simulink library "acc"  (R2021b)
settings: Solver=VariableStepAuto  StartTime=0.0  StopTime=10.0  RelTol=1e-3
undefined symbols (not defined in the file or in its folder): AACC_CondensorFanReq_X_enum, AACC_EWP1CCUReq_X_C, AACC_EWP1EDUReq_X_C, AACC_EWP1HVBReq_X_C, AACC_EWP2CCUReq_X_C, AACC_EWP2EDUReq_X_C, AACC_EWP2HVBReq_X_C, AACC_FWV1CCUReq_X_C, AACC_FWV1EDUReq_X_C, AACC_FWV1HVBReq_X_C, AACC_FWV2CCUReq_X_C, AACC_FWV2EDUReq_X_C, AACC_FWV2HVBReq_X_C, AACC_TWVCCUReq_X_C, AACC_TWVEDUReq_X_C, AACC_TWVHVBReq_X_C, ENUM_ACCMODE_CHARGING, ENUM_ACCMODE_COOLING, ENUM_ACCMODE_OFF, ENUM_ACCMODE_SERVICE, ENUM_ACREQ_COOLING, ENUM_ACREQ_NOREQUEST, ENUM_CHILLERINITREQ_NONE, ENUM_CHILLERINITREQ_START, ENUM_CHILLERINITREQ_WAITING, ENUM_CHILLERINITSTA_FINISH, ENUM_CHILLERINITSTA_INPROCESS, ENUM_COOLFANREQ_HI, ENUM_COOLFANREQ_LOW, ENUM_COOLFANREQ_OFF, ENUM_LVBATTSTA_FAIL, ENUM_LVBATTSTA_NORMAL, ENUM_PMMMODE_CHARGE, ENUM_PMMMODE_DRIVE, ENUM_PMMMODE_LVBATCHRG, ENUM_PMMMODE_POWERUP, ENUM_THCMSYS_INACTIVE, FALSE, KACC_CCUFanHighOffTemp_C, KACC_CCUFanHighOnTemp_C, KACC_CCUFanLowOffTemp_C, KACC_CCUFanLowOnTemp_C, KACC_ChillerInitTime_s, KACC_ChillerStartTime_s, KACC_DCDCCalPwrAvailRsv_kW, KACC_EDUFanHighOffTemp_C, KACC_EDUFanHighOnTemp_C, KACC_EDUFanLowOffTemp_C, KACC_EDUFanLowOnTemp_C, KACC_EWP1CalDutyVal_pct, KACC_EWP1CalON_flg, KACC_EWP2CalDutyVal_pct, KACC_EWP2CalON_flg, KACC_EXVCalON_flg, KACC_EXVCalVal_cnt, KACC_FanCalON_flg, KACC_FanCalVal_enum, KACC_FWV1CalON_flg, KACC_FWV1CalVal_flg, KACC_FWV2CalON_flg ... (+51)
libraries: simulink x1
(part 1 of 2)
settings Model: Creator=13615  LastModifiedBy=FVT23131
settings SolverCC: AlgebraicLoopSolver=TrustRegion
settings DataIOCC: SaveFormat=Array  SignalLoggingSaveFormat=ModelDataLogs  ReturnWorkspaceOutputs=off
settings OptimizationCC: BlockReduction=off  BooleanDataType=off
settings DebuggingCC: SaveWithParameterizedLinksMsg=none  UnderspecifiedInitializationDetection=Classic  MergeDetectMultiDrivingBlocksExec=none  SignalResolutionControl=TryResolveAllWithWarning  SFMachineParentedDataDiag=warning  ArithmeticOperatorsInVariantConditions=warning
settings HardwareCC: TargetUnknown=on
settings ModelReferenceCC: PropagateSignalLabelsOutOfModel=off
settings SFSimCC: CustomCodeUndefinedFunction=UseInterfaceOnly
settings ConfigComp: CovMetricSettings=dw  CovSaveCumulativeToWorkspaceVar=on  CovSaveSingleToWorkspaceVar=on

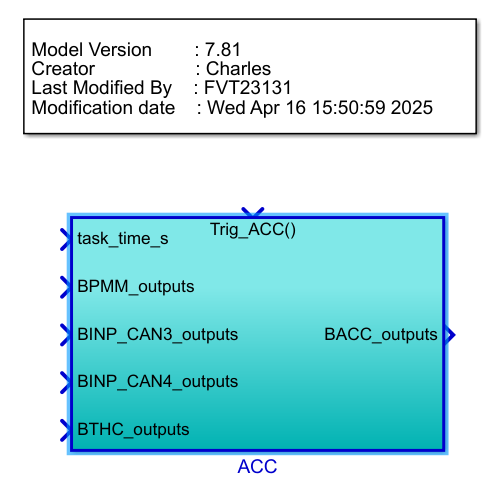
[thumbnail: Simulink's stored preview of the top-level diagram]
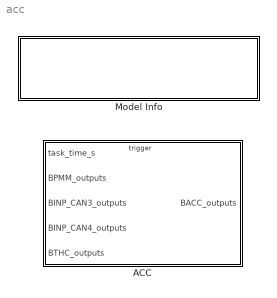
== system acc ==
  ACC : Subsystem  TreatAsAtomicUnit=on
      settings: RTWSystemCode=Nonreusable function  RTWFcnNameOpts=Use subsystem name  RTWFileNameOpts=Use subsystem name
  Model Info : Subsystem  LoadFcn=slcm LoadBlock;  InitFcn=slcm('UpdateAllCMBlocksInThisModelInit')  mask(CMBlock){InitialSaveTempField=, InitialBlockCM=None, BlockCM=None, Frame=on, SaveTempField=, DisplayStringWithTags=|, MaskDisplayString=Model Version        : 7.84\nCreator                   : Charles\nLast Modified By    : FVT23131\nModification date    : Wed Apr 16 17:01:18 2025, HorizontalTextAlignment=Left, LeftAlignmentValue=0.02, SourceBlockDiagram=acc, TagMaxNumber=20, CMTag1=, CMTag2=, CMTag3=, CMTag4=, CMTag5=, CMTag6=, CMTag7=, CMTag8=, CMTag9=, CMTag10=, CMTag11=, CMTag12=, CMTag13=, CMTag14=, CMTag15=, CMTag16=, CMTag17=, CMTag18=, CMTag19=, CMTag20=}
      mask DisplayStringWithTags=|
      | Model Version        : %<ModelVersion>
      | Creator                   : Charles
      | Last Modified By    : %<LastModifiedBy>
      | Modification date    : %<LastModificationDate>
      mask help: This block allows revision control information to be displayed within the model.
      settings: CopyFcn=slcm CopyBlock;  DeleteFcn=slcm Cancel;  PostSaveFcn=slcm('UpdateAllCMBlocksInThisModel')  NameChangeFcn=slcm Rename;  OpenFcn=slcm
      mask Display: text(str2num(LeftAlignmentValue), 0.5, MaskDisplayString, 'HorizontalAlignment', HorizontalTextAlignment)

== system acc/ACC ==
  task_time_s : Inport
  BPMM_outputs : Inport  Port=2  OutDataTypeStr=Bus: BPMM_outputs
  BINP_CAN3_outputs : Inport  Port=3  OutDataTypeStr=Bus: BINP_CAN3_outputs
  BINP_CAN4_outputs : Inport  Port=4  OutDataTypeStr=Bus: BINP_CAN4_outputs
  BTHC_outputs : Inport  Port=5  OutDataTypeStr=Bus: BTHC_outputs
  Trig_ACC : TriggerPort  TriggerType=function-call  VariantControl=(inherit)
  ACC : Subsystem  Commented=on  AncestorBlock=acc/ACC/ACC
  Bus Creator : BusCreator  Inputs=4  OutDataTypeStr=Bus: BACC_outputs
  Bus Selector : BusSelector  OutputSignals=VINP_COMPActualPwr_W
  Bus Selector1 : BusSelector  OutputSignals=VINP_LVBattDet12V_V,VINP_HVBPwrAvailDchrg_kW,VINP_FrMCUDCBusVolt_V,VINP_FrMCUDCBusCurr_A,VINP_RrMCUDCBusVolt_V,VINP_RrMCUDCBusCurr_A,VINP_DCDCHVCur_A,VINP_DCDCInVoltInf_V
  Bus Selector12 : BusSelector  OutputSignals=VTHC_FDFrLeAPTCHeatPwrCmd_W,VTHC_FDFrRiAPTCHeatPwrCmd_W,VTHC_FDRrAPTCHeatPwrCmd_W,VTHC_FDFrWPTCHeatPwrCmd_W
  Bus Selector2 : BusSelector  OutputSignals=VPMM_HVPwrSta_flg,VPMM_LVPwrSta_flg
  Model Info : simulink/Model-Wide Utilities/Model Info  Frame=on  DisplayStringWithTags=|  HorizontalTextAlignment=Center  LeftAlignmentValue=0.5
      | $Id: ACC.mdl 2018-05-29 Lon $
      | Modified By %<ModifiedBy>
      | Modified Date : %<ModifiedDate>
  THCM : Subsystem
  BACC_outputs : Outport  OutDataTypeStr=Bus: BACC_outputs  VectorParamsAs1DForOutWhenUnconnected=off
  wires:
  BPMM_outputs/1 -> Bus Selector2/1
  Bus Creator/1 -> BACC_outputs/1  "BACC_outputs"
  BINP_CAN3_outputs/1 -> Bus Selector1/1
  Bus Selector1/1 -> THCM/4(VINP_LVBattDet12V_V)  "<VINP_LVBattDet12V_V>"
  task_time_s/1 -> THCM/1(task_time_s)
  Bus Selector1/2 -> THCM/5(VINP_HVBPwrAvailDchrg_kW)  "<VINP_HVBPwrAvailDchrg_kW>"
  Bus Selector1/3 -> THCM/6(VINP_FrMCUDCBusVolt_V)  "<VINP_FrMCUDCBusVolt_V>"
  Bus Selector1/4 -> THCM/7(VINP_FrMCUDCBusCurr_A)  "<VINP_FrMCUDCBusCurr_A>"
  Bus Selector1/5 -> THCM/8(VINP_RrMCUDCBusVolt_V)  "<VINP_RrMCUDCBusVolt_V>"
  Bus Selector1/6 -> THCM/9(VINP_RrMCUDCBusCurr_A)  "<VINP_RrMCUDCBusCurr_A>"
  THCM/3(VACC_VehHVPwrAvail4THCM_W) -> Bus Creator/3
  THCM/1(VACC_HVTHCMSysAvail_enum) -> Bus Creator/1
  THCM/2(VACC_LVBattVoltSta_enum) -> Bus Creator/2
  Bus Selector2/1 -> THCM/2(VPMM_HVPwrSta_flg)  "<VPMM_HVPwrSta_flg>"
  Bus Selector2/2 -> THCM/3(VPMM_LVPwrSta_flg)  "<VPMM_LVPwrSta_flg>"
  Bus Selector1/7 -> THCM/10(VINP_DCDCHVCur_A)  "<VINP_DCDCHVCur_A>"
  Bus Selector1/8 -> THCM/11(VINP_DCDCInVoltInf_V)  "<VINP_DCDCInVoltInf_V>"
  BINP_CAN4_outputs/1 -> Bus Selector/1
  Bus Selector/1 -> THCM/12(VINP_COMPActualPwr_W)  "<VINP_COMPActualPwr_W>"
  BTHC_outputs/1 -> Bus Selector12/1
  Bus Selector12/1 -> THCM/13(VTHC_FDFrLeAPTCHeatPwrCmd_W)  "<VTHC_FDFrLeAPTCHeatPwrCmd_W>"
  Bus Selector12/2 -> THCM/14(VTHC_FDFrRiAPTCHeatPwrCmd_W)  "<VTHC_FDFrRiAPTCHeatPwrCmd_W>"
  Bus Selector12/3 -> THCM/15(VTHC_FDRrAPTCHeatPwrCmd_W)  "<VTHC_FDRrAPTCHeatPwrCmd_W>"
  Bus Selector12/4 -> THCM/16(VTHC_FDFrWPTCHeatPwrCmd_W)  "<VTHC_FDFrWPTCHeatPwrCmd_W>"
  THCM/4(VACC_TMPwrAvailDchrg_kW) -> Bus Creator/4

== system acc/Model Info ==
  EmptySubsystem : Subsystem

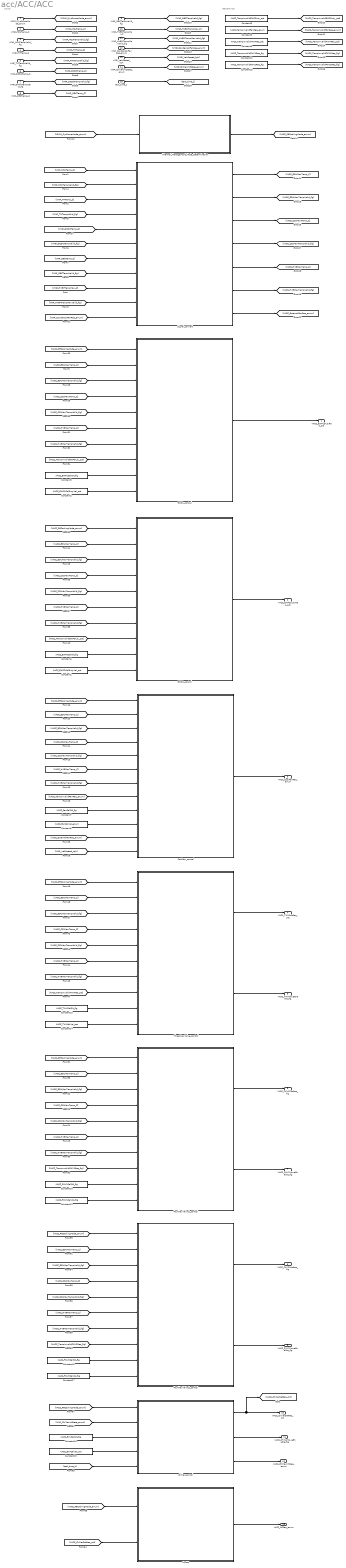
== system acc/ACC/ACC ==
  note: General Cal
  note: Inputs
  VPMM_SysPowerMode_enum : Inport
  VINP_MCUTemp_C : Inport  Port=2
  VINP_MCUTempValid_flg : Inport  Port=3
  VINP_TMTemp_C : Inport  Port=4
  VINP_TMTempValid_flg : Inport  Port=5
  VINP_DCDCTemp_C : Inport  Port=6
  VINP_DCDCTempValid_flg : Inport  Port=7
  VINP_OBCTemp_C : Inport  Port=8
  VINP_OBCTempValid_flg : Inport  Port=9
  VINP_HVBMTempMax_C : Inport  Port=10
  VINP_HVBMTempMaxValid_flg : Inport  Port=11
  VINP_CondensorFanReq_enum : Inport  Port=12
  VINP_VehSpeed_kph : Inport  Port=13
  VINP_ChillerInitState_enum : Inport  Port=14
  task_time_s : Inport  Port=15
  ACReq : Subsystem
  Chiller_control : Subsystem
  Constant1 : Constant  Value=KACC_EWP2CalDutyVal_pct
  Constant10 : Constant  Value=KACC_FWV1CalON_flg
  Constant11 : Constant  Value=KACC_FWV1CalVal_flg
  Constant12 : Constant  Value=KACC_TempInvalidFWV1Req_flg
  Constant13 : Constant  Value=KACC_TWVCalON_flg
  Constant14 : Constant  Value=KACC_TWVCalVal_pct
  Constant15 : Constant  Value=KACC_TempInvalidFWV2Req_flg
  Constant16 : Constant  Value=KACC_FWV2CalON_flg
  Constant17 : Constant  Value=KACC_FWV2CalVal_flg
  Constant18 : Constant  Value=KACC_EXVCalON_flg
  Constant19 : Constant  Value=KACC_EXVCalVal_cnt
  Constant2 : Constant  Value=KACC_EWP1CalDutyVal_pct
  Constant3 : Constant  Value=KACC_EWP1CalON_flg
  Constant4 : Constant  Value=KACC_EWP2CalON_flg
  Constant5 : Constant  Value=KACC_TempInvalidEWPDuty_pct
  Constant6 : Constant  Value=KACC_FanCalVal_enum
  Constant7 : Constant  Value=KACC_FanCalON_flg
  Constant8 : Constant  Value=KACC_TempInvalidTWVReq_pct
  Constant9 : Constant  Value=KACC_TempInvalidFanReq_enum
  CoolFan_control : Subsystem
  EWP1_control : Subsystem
  EWP2_control : Subsystem
  FourWayValve1_control : Subsystem
  FourWayValve2_control : Subsystem
  Signal_convert : Subsystem
  Thermal_Managemant_Mode_Determination : Subsystem
  ThreeWayValve_control : Subsystem
  VACC_EWP1DutyReq_pct : Outport  VectorParamsAs1DForOutWhenUnconnected=off
  VACC_EWP2DutyReq_pct : Outport  Port=2  VectorParamsAs1DForOutWhenUnconnected=off
  VACC_CoolFanReq_enum : Outport  Port=3  VectorParamsAs1DForOutWhenUnconnected=off
  VACC_TWVPosReq_pct : Outport  Port=4  VectorParamsAs1DForOutWhenUnconnected=off
  VACC_TWVMoveEnable_flg : Outport  Port=5  VectorParamsAs1DForOutWhenUnconnected=off
  VACC_FWV1PosReq_flg : Outport  Port=6  VectorParamsAs1DForOutWhenUnconnected=off
  VACC_FWV1MoveEnable_flg : Outport  Port=7  VectorParamsAs1DForOutWhenUnconnected=off
  VACC_FWV2PosReq_flg : Outport  Port=8  VectorParamsAs1DForOutWhenUnconnected=off
  VACC_FWV2MoveEnable_flg : Outport  Port=9  VectorParamsAs1DForOutWhenUnconnected=off
  VACC_ChillerSetReq_cnt : Outport  Port=10  VectorParamsAs1DForOutWhenUnconnected=off
  VACC_ChillerMoveEnable_flg : Outport  Port=11  VectorParamsAs1DForOutWhenUnconnected=off
  VACC_ChillerInitReq_enum : Outport  Port=12  VectorParamsAs1DForOutWhenUnconnected=off
  VACC_ACReq_enum : Outport  Port=13  VectorParamsAs1DForOutWhenUnconnected=off
  wires:
  [task_time_s] -> Chiller_control/5(task_time_s)
  task_time_s/1 -> [task_time_s]
  [VINP_ChillerInitState_enum] -> Chiller_control/2(VINP_ChillerInitState_enum)
  VINP_ChillerInitState_enum/1 -> [VINP_ChillerInitState_enum]
  Chiller_control/3(VACC_ChillerInitReq_enum) -> VACC_ChillerInitReq_enum/1  "VACC_ChillerInitReq_enum"
  Chiller_control/1(VACC_ChillerSetReq_cnt) -> [VACC_ChillerSetReq_cnt], VACC_ChillerSetReq_cnt/1  "VACC_ChillerSetReq_cnt"
  [VACC_PECoolingMode_enum] -> Chiller_control/1(VACC_PECoolingMode_enum)
  Constant18/1 -> Chiller_control/3(KACC_EXVCalON_flg)  "KACC_EXVCalON_flg"
  Constant19/1 -> Chiller_control/4(KACC_EXVCalVal_cnt)  "KACC_EXVCalVal_cnt"
  Chiller_control/2(VACC_ChillerMoveEnable_flg) -> VACC_ChillerMoveEnable_flg/1  "VACC_ChillerMoveEnable_flg"
  FourWayValve2_control/2(VACC_FWV2MoveEnable_flg) -> VACC_FWV2MoveEnable_flg/1  "VACC_FWV2MoveEnable_flg"
  Constant17/1 -> FourWayValve2_control/10(KACC_FWV2CalVal_flg)  "KACC_FWV2CalVal_flg"
  Constant16/1 -> FourWayValve2_control/9(KACC_FWV2CalON_flg)  "KACC_FWV2CalON_flg"
  [VACC_PECoolingMode_enum] -> FourWayValve2_control/1(VACC_PECoolingMode_enum)
  [VACC_CCUMaxTempValid_flg] -> FourWayValve2_control/5(VACC_CCUMaxTempValid_flg)
  [VACC_CCUMaxTemp_C] -> FourWayValve2_control/4(VACC_CCUMaxTemp_C)
  [VACC_EDUMaxTemp_C] -> FourWayValve2_control/2(VACC_EDUMaxTemp_C)
  [VACC_EDUMaxTempValid_flg] -> FourWayValve2_control/3(VACC_EDUMaxTempValid_flg)
  [VACC_HVBMaxTempValid_flg] -> FourWayValve2_control/7(VACC_HVBMaxTempValid_flg)
  FourWayValve2_control/1(VACC_FWV2PosReq_flg) -> VACC_FWV2PosReq_flg/1  "VACC_FWV2PosReq_flg"
  [VACC_HVBMaxTemp_C] -> FourWayValve2_control/6(VACC_HVBMaxTemp_C)
  [KACC_TempInvalidFWV2Req_flg] -> FourWayValve2_control/8(KACC_TempInvalidFWV2Req_flg)
  [KACC_TempInvalidFWV1Req_flg] -> FourWayValve1_control/8(KACC_TempInvalidFWV1Req_flg)
  [KACC_TempInvalidTWVReq_pct] -> ThreeWayValve_control/8(KACC_TempInvalidTWVReq_pct)
  Constant15/1 -> [KACC_TempInvalidFWV2Req_flg]  "KACC_TempInvalidFWV2Req_flg"
  Constant12/1 -> [KACC_TempInvalidFWV1Req_flg]  "KACC_TempInvalidFWV1Req_flg"
  [VACC_HVBMaxTemp_C] -> FourWayValve1_control/6(VACC_HVBMaxTemp_C)
  FourWayValve1_control/1(VACC_FWV1PosReq_flg) -> VACC_FWV1PosReq_flg/1  "VACC_FWV1PosReq_flg"
  [VACC_HVBMaxTempValid_flg] -> FourWayValve1_control/7(VACC_HVBMaxTempValid_flg)
  [VACC_EDUMaxTempValid_flg] -> FourWayValve1_control/3(VACC_EDUMaxTempValid_flg)
  [VACC_EDUMaxTemp_C] -> FourWayValve1_control/2(VACC_EDUMaxTemp_C)
  [VACC_CCUMaxTemp_C] -> FourWayValve1_control/4(VACC_CCUMaxTemp_C)
  [VACC_CCUMaxTempValid_flg] -> FourWayValve1_control/5(VACC_CCUMaxTempValid_flg)
  [VACC_PECoolingMode_enum] -> FourWayValve1_control/1(VACC_PECoolingMode_enum)
  Constant10/1 -> FourWayValve1_control/9(KACC_FWV1CalON_flg)  "KACC_FWV1CalON_flg"
  Constant11/1 -> FourWayValve1_control/10(KACC_FWV1CalVal_flg)  "KACC_FWV1CalVal_flg"
  FourWayValve1_control/2(VACC_FWV1MoveEnable_flg) -> VACC_FWV1MoveEnable_flg/1  "VACC_FWV1MoveEnable_flg"
  ThreeWayValve_control/2(VACC_TWVMoveEnable_flg) -> VACC_TWVMoveEnable_flg/1  "VACC_TWVMoveEnable_flg"
  Constant14/1 -> ThreeWayValve_control/10(KACC_TWVCalVal_pct)  "KACC_TWVCalVal_pct"
  Constant13/1 -> ThreeWayValve_control/9(KACC_TWVCalON_flg)  "KACC_TWVCalON_flg"
  Constant8/1 -> [KACC_TempInvalidTWVReq_pct]  "KACC_TempInvalidTWVReq_pct"
  [VACC_PECoolingMode_enum] -> ThreeWayValve_control/1(VACC_PECoolingMode_enum)
  [VACC_CCUMaxTempValid_flg] -> ThreeWayValve_control/5(VACC_CCUMaxTempValid_flg)
  [VACC_CCUMaxTemp_C] -> ThreeWayValve_control/4(VACC_CCUMaxTemp_C)
  [VACC_EDUMaxTemp_C] -> ThreeWayValve_control/2(VACC_EDUMaxTemp_C)
  [VACC_EDUMaxTempValid_flg] -> ThreeWayValve_control/3(VACC_EDUMaxTempValid_flg)
  [VACC_HVBMaxTempValid_flg] -> ThreeWayValve_control/7(VACC_HVBMaxTempValid_flg)
  ThreeWayValve_control/1(VACC_TWVPosReq_pct) -> VACC_TWVPosReq_pct/1  "VACC_TWVPosReq_pct"
  [VACC_HVBMaxTemp_C] -> ThreeWayValve_control/6(VACC_HVBMaxTemp_C)
  [VINP_VehSpeed_kph] -> CoolFan_control/12(VINP_VehSpeed_kph)
  VINP_VehSpeed_kph/1 -> [VINP_VehSpeed_kph]
  [VACC_ExternalFanReq_enum] -> CoolFan_control/11(VACC_ExternalFanReq_enum)
  Signal_convert/7(VACC_ExternalFanReq_enum) -> [VACC_ExternalFanReq_enum]  "VACC_ExternalFanReq_enum"
  [VINP_CondensorFanReq_enum] -> Signal_convert/11(VINP_CondensorFanReq_enum)
  [KACC_TempInvalidFanReq_enum] -> CoolFan_control/8(KACC_TempInvalidFanReq_enum)
  Constant6/1 -> CoolFan_control/10(KACC_FanCalVal_enum)  "KACC_FanCalVal_enum"
  Constant7/1 -> CoolFan_control/9(KACC_FanCalON_flg)  "KACC_FanCalON_flg"
  [VACC_CCUMaxTemp_C] -> CoolFan_control/4(VACC_CCUMaxTemp_C)
  [VACC_EDUMaxTempValid_flg] -> CoolFan_control/3(VACC_EDUMaxTempValid_flg)
  [VACC_EDUMaxTemp_C] -> CoolFan_control/2(VACC_EDUMaxTemp_C)
  [VACC_HVBMaxTempValid_flg] -> CoolFan_control/7(VACC_HVBMaxTempValid_flg)
  [VACC_HVBMaxTemp_C] -> CoolFan_control/6(VACC_HVBMaxTemp_C)
  [VACC_CCUMaxTempValid_flg] -> CoolFan_control/5(VACC_CCUMaxTempValid_flg)
  [VACC_PECoolingMode_enum] -> CoolFan_control/1(VACC_PECoolingMode_enum)
  CoolFan_control/1(VACC_CoolFanReq_enum) -> VACC_CoolFanReq_enum/1  "VACC_CoolFanReq_enum"
  EWP2_control/1(VACC_EWP2DutyReq_pct) -> VACC_EWP2DutyReq_pct/1  "VACC_EWP2DutyReq_pct"
  [VACC_PECoolingMode_enum] -> EWP2_control/1(VACC_PECoolingMode_enum)
  [VACC_CCUMaxTempValid_flg] -> EWP2_control/5(VACC_CCUMaxTempValid_flg)
  [VACC_HVBMaxTemp_C] -> EWP2_control/6(VACC_HVBMaxTemp_C)
  [VACC_HVBMaxTempValid_flg] -> EWP2_control/7(VACC_HVBMaxTempValid_flg)
  [VACC_EDUMaxTemp_C] -> EWP2_control/2(VACC_EDUMaxTemp_C)
  [VACC_EDUMaxTempValid_flg] -> EWP2_control/3(VACC_EDUMaxTempValid_flg)
  [VACC_CCUMaxTemp_C] -> EWP2_control/4(VACC_CCUMaxTemp_C)
  [KACC_TempInvalidEWPDuty_pct] -> EWP2_control/8(KACC_TempInvalidEWPDuty_pct)
  Constant4/1 -> EWP2_control/9(KACC_EWP2CalON_flg)  "KACC_EWP2CalON_flg"
  Constant1/1 -> EWP2_control/10(KACC_EWP2CalDutyVal_pct)  "KACC_EWP2CalDutyVal_pct"
  Constant2/1 -> EWP1_control/10(KACC_EWP1CalDutyVal_pct)  "KACC_EWP1CalDutyVal_pct"
  Constant3/1 -> EWP1_control/9(KACC_EWP1CalON_flg)  "KACC_EWP1CalON_flg"
  [KACC_TempInvalidEWPDuty_pct] -> EWP1_control/8(KACC_TempInvalidEWPDuty_pct)
  [VACC_CCUMaxTemp_C] -> EWP1_control/4(VACC_CCUMaxTemp_C)
  [VACC_EDUMaxTempValid_flg] -> EWP1_control/3(VACC_EDUMaxTempValid_flg)
  [VACC_EDUMaxTemp_C] -> EWP1_control/2(VACC_EDUMaxTemp_C)
  [VACC_HVBMaxTempValid_flg] -> EWP1_control/7(VACC_HVBMaxTempValid_flg)
  [VACC_HVBMaxTemp_C] -> EWP1_control/6(VACC_HVBMaxTemp_C)
  [VACC_CCUMaxTempValid_flg] -> EWP1_control/5(VACC_CCUMaxTempValid_flg)
  [VACC_PECoolingMode_enum] -> EWP1_control/1(VACC_PECoolingMode_enum)
  Constant9/1 -> [KACC_TempInvalidFanReq_enum]  "KACC_TempInvalidFanReq_enum"
  Constant5/1 -> [KACC_TempInvalidEWPDuty_pct]  "KACC_TempInvalidEWPDuty_pct"
  Signal_convert/4(VACC_CCUMaxTempValid_flg) -> [VACC_CCUMaxTempValid_flg]  "VACC_CCUMaxTempValid_flg"
  Signal_convert/5(VACC_HVBMaxTemp_C) -> [VACC_HVBMaxTemp_C]  "VACC_HVBMaxTemp_C"
  Signal_convert/3(VACC_CCUMaxTemp_C) -> [VACC_CCUMaxTemp_C]  "VACC_CCUMaxTemp_C"
  Signal_convert/6(VACC_HVBMaxTempValid_flg) -> [VACC_HVBMaxTempValid_flg]  "VACC_HVBMaxTempValid_flg"
  Signal_convert/2(VACC_EDUMaxTempValid_flg) -> [VACC_EDUMaxTempValid_flg]  "VACC_EDUMaxTempValid_flg"
  Signal_convert/1(VACC_EDUMaxTemp_C) -> [VACC_EDUMaxTemp_C]  "VACC_EDUMaxTemp_C"
  [VINP_HVBMTempMaxValid_flg] -> Signal_convert/10(VINP_HVBMTempMaxValid_flg)
  [VINP_HVBMTempMax_C] -> Signal_convert/9(VINP_HVBMTempMax_C)
  [VINP_OBCTempValid_flg] -> Signal_convert/8(VINP_OBCTempValid_flg)
  [VINP_OBCTemp_C] -> Signal_convert/7(VINP_OBCTemp_C)
  [VINP_MCUTemp_C] -> Signal_convert/1(VINP_MCUTemp_C)
  [VINP_DCDCTempValid_flg] -> Signal_convert/6(VINP_DCDCTempValid_flg)
  [VINP_MCUTempValid_flg] -> Signal_convert/2(VINP_MCUTempValid_flg)
  [VINP_TMTemp_C] -> Signal_convert/3(VINP_TMTemp_C)
  [VINP_TMTempValid_flg] -> Signal_convert/4(VINP_TMTempValid_flg)
  [VINP_DCDCTemp_C] -> Signal_convert/5(VINP_DCDCTemp_C)
  VINP_CondensorFanReq_enum/1 -> [VINP_CondensorFanReq_enum]
  VINP_DCDCTemp_C/1 -> [VINP_DCDCTemp_C]
  VINP_TMTemp_C/1 -> [VINP_TMTemp_C]
  VINP_MCUTemp_C/1 -> [VINP_MCUTemp_C]
  VPMM_SysPowerMode_enum/1 -> [VPMM_SysPowerMode_enum]
  VINP_OBCTemp_C/1 -> [VINP_OBCTemp_C]
  VINP_HVBMTempMax_C/1 -> [VINP_HVBMTempMax_C]
  VINP_MCUTempValid_flg/1 -> [VINP_MCUTempValid_flg]
  VINP_TMTempValid_flg/1 -> [VINP_TMTempValid_flg]
  VINP_DCDCTempValid_flg/1 -> [VINP_DCDCTempValid_flg]
  VINP_OBCTempValid_flg/1 -> [VINP_OBCTempValid_flg]
  VINP_HVBMTempMaxValid_flg/1 -> [VINP_HVBMTempMaxValid_flg]
  Thermal_Managemant_Mode_Determination/1(VACC_PECoolingMode_enum) -> [VACC_PECoolingMode_enum]
  [VPMM_SysPowerMode_enum] -> Thermal_Managemant_Mode_Determination/1(VPMM_SysPowerMode_enum)
  EWP1_control/1(VACC_EWP1DutyReq_pct) -> VACC_EWP1DutyReq_pct/1  "VACC_EWP1DutyReq_pct"
  [VACC_ChillerSetReq_cnt] -> ACReq/2(VACC_ChillerSetReq_cnt)
  [VACC_PECoolingMode_enum] -> ACReq/1(VACC_PECoolingMode_enum)
  ACReq/1(VACC_ACReq_enum) -> VACC_ACReq_enum/1  "VACC_ACReq_enum"

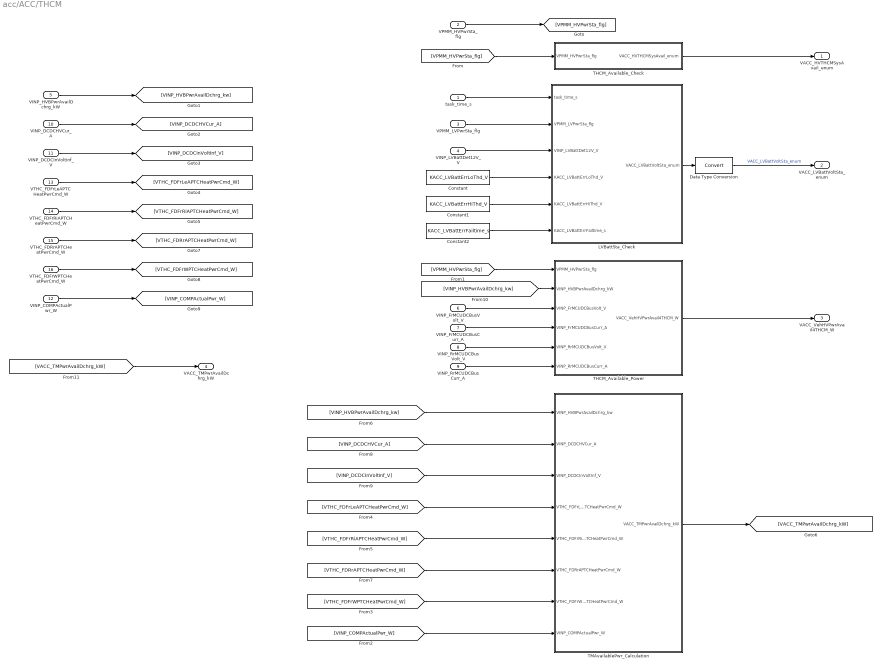
== system acc/ACC/THCM ==
  task_time_s : Inport
  VPMM_HVPwrSta_flg : Inport  Port=2
  VPMM_LVPwrSta_flg : Inport  Port=3
  VINP_LVBattDet12V_V : Inport  Port=4
  VINP_HVBPwrAvailDchrg_kW : Inport  Port=5
  VINP_FrMCUDCBusVolt_V : Inport  Port=6
  VINP_FrMCUDCBusCurr_A : Inport  Port=7
  VINP_RrMCUDCBusVolt_V : Inport  Port=8
  VINP_RrMCUDCBusCurr_A : Inport  Port=9
  VINP_DCDCHVCur_A : Inport  Port=10
  VINP_DCDCInVoltInf_V : Inport  Port=11
  VINP_COMPActualPwr_W : Inport  Port=12
  VTHC_FDFrLeAPTCHeatPwrCmd_W : Inport  Port=13
  VTHC_FDFrRiAPTCHeatPwrCmd_W : Inport  Port=14
  VTHC_FDRrAPTCHeatPwrCmd_W : Inport  Port=15
  VTHC_FDFrWPTCHeatPwrCmd_W : Inport  Port=16
  Constant : Constant  Value=KACC_LVBattErrLoThd_V
  Constant1 : Constant  Value=KACC_LVBattErrHiThd_V
  Constant2 : Constant  Value=KACC_LVBattErrFailtime_s
  Data Type Conversion : DataTypeConversion
  LVBattSta_Check : Stateflow chart  TreatAsAtomicUnit=on
  THCM_Available_Check : Subsystem
  THCM_Available_Power : Subsystem
  TMAvailablePwr_Calculation : Subsystem
  VACC_HVTHCMSysAvail_enum : Outport
  VACC_LVBattVoltSta_enum : Outport  Port=2
  VACC_VehHVPwrAvail4THCM_W : Outport  Port=3
  VACC_TMPwrAvailDchrg_kW : Outport  Port=4
  wires:
  VINP_LVBattDet12V_V/1 -> LVBattSta_Check/3(VINP_LVBattDet12V_V)
  Constant/1 -> LVBattSta_Check/4(KACC_LVBattErrLoThd_V)
  Constant1/1 -> LVBattSta_Check/5(KACC_LVBattErrHiThd_V)
  Constant2/1 -> LVBattSta_Check/6(KACC_LVBattErrFailtime_s)
  LVBattSta_Check/1(VACC_LVBattVoltSta_enum) -> Data Type Conversion/1
  task_time_s/1 -> LVBattSta_Check/1(task_time_s)
  VPMM_HVPwrSta_flg/1 -> [VPMM_HVPwrSta_flg]
  Data Type Conversion/1 -> VACC_LVBattVoltSta_enum/1  "VACC_LVBattVoltSta_enum"
  VPMM_LVPwrSta_flg/1 -> LVBattSta_Check/2(VPMM_LVPwrSta_flg)
  [VPMM_HVPwrSta_flg] -> THCM_Available_Check/1(VPMM_HVPwrSta_flg)
  THCM_Available_Check/1(VACC_HVTHCMSysAvail_enum) -> VACC_HVTHCMSysAvail_enum/1
  [VPMM_HVPwrSta_flg] -> THCM_Available_Power/1(VPMM_HVPwrSta_flg)
  THCM_Available_Power/1(VACC_VehHVPwrAvail4THCM_W) -> VACC_VehHVPwrAvail4THCM_W/1
  VINP_FrMCUDCBusVolt_V/1 -> THCM_Available_Power/3(VINP_FrMCUDCBusVolt_V)
  VINP_FrMCUDCBusCurr_A/1 -> THCM_Available_Power/4(VINP_FrMCUDCBusCurr_A)
  VINP_RrMCUDCBusVolt_V/1 -> THCM_Available_Power/5(VINP_RrMCUDCBusVolt_V)
  VINP_RrMCUDCBusCurr_A/1 -> THCM_Available_Power/6(VINP_RrMCUDCBusCurr_A)
  [VINP_HVBPwrAvailDchrg_kw] -> THCM_Available_Power/2(VINP_HVBPwrAvailDchrg_kW)
  [VINP_HVBPwrAvailDchrg_kw] -> TMAvailablePwr_Calculation/1(VINP_HVBPwrAvailDchrg_kw)
  TMAvailablePwr_Calculation/1(VACC_TMPwrAvailDchrg_kW) -> [VACC_TMPwrAvailDchrg_kW]
  [VTHC_FDFrWPTCHeatPwrCmd_W] -> TMAvailablePwr_Calculation/7(VTHC_FDFrWPTCHeatPwrCmd_W)
  [VTHC_FDRrAPTCHeatPwrCmd_W] -> TMAvailablePwr_Calculation/6(VTHC_FDRrAPTCHeatPwrCmd_W)
  [VTHC_FDFrLeAPTCHeatPwrCmd_W] -> TMAvailablePwr_Calculation/4(VTHC_FDFrLeAPTCHeatPwrCmd_W)
  [VINP_DCDCInVoltInf_V] -> TMAvailablePwr_Calculation/3(VINP_DCDCInVoltInf_V)
  [VTHC_FDFrRiAPTCHeatPwrCmd_W] -> TMAvailablePwr_Calculation/5(VTHC_FDFrRiAPTCHeatPwrCmd_W)
  [VINP_COMPActualPwr_W] -> TMAvailablePwr_Calculation/8(VINP_COMPActualPwr_W)
  VINP_HVBPwrAvailDchrg_kW/1 -> [VINP_HVBPwrAvailDchrg_kw]
  VINP_DCDCHVCur_A/1 -> [VINP_DCDCHVCur_A]
  VINP_DCDCInVoltInf_V/1 -> [VINP_DCDCInVoltInf_V]
  VTHC_FDFrLeAPTCHeatPwrCmd_W/1 -> [VTHC_FDFrLeAPTCHeatPwrCmd_W]
  VTHC_FDFrRiAPTCHeatPwrCmd_W/1 -> [VTHC_FDFrRiAPTCHeatPwrCmd_W]
  VTHC_FDRrAPTCHeatPwrCmd_W/1 -> [VTHC_FDRrAPTCHeatPwrCmd_W]
  VTHC_FDFrWPTCHeatPwrCmd_W/1 -> [VTHC_FDFrWPTCHeatPwrCmd_W]
  VINP_COMPActualPwr_W/1 -> [VINP_COMPActualPwr_W]
  [VACC_TMPwrAvailDchrg_kW] -> VACC_TMPwrAvailDchrg_kW/1
  [VINP_DCDCHVCur_A] -> TMAvailablePwr_Calculation/2(VINP_DCDCHVCur_A)

== system acc/Model Info/EmptySubsystem ==

== system acc/ACC/ACC/ACReq ==
  VACC_PECoolingMode_enum : Inport
  VACC_ChillerSetReq_cnt : Inport  Port=2
  Constant1 : Constant  Value=ZERO_INT
  Constant10 : Constant  Value=ENUM_ACCMODE_CHARGING
  Constant11 : Constant  Value=ENUM_ACCMODE_COOLING
  Constant2 : Constant  Value=ENUM_ACREQ_COOLING
  Constant3 : Constant  Value=ENUM_ACREQ_NOREQUEST
  OR2 : Logic  Operator=OR  AllPortsSameDT=off  OutDataTypeStr=boolean
  OR3 : Logic  AllPortsSameDT=off  OutDataTypeStr=boolean
  Relational Operator1 : RelationalOperator  Operator===  OutDataTypeStr=boolean  RndMeth=Simplest
  Relational Operator2 : RelationalOperator  Operator=>  OutDataTypeStr=boolean  RndMeth=Simplest
  Relational Operator3 : RelationalOperator  Operator===  OutDataTypeStr=boolean  RndMeth=Simplest
  Switch2 : Switch  Criteria=u2 ~= 0
      settings: AttributesFormatString=%<Criteria>
  VACC_ACReq_enum : Outport
  wires:
  VACC_ChillerSetReq_cnt/1 -> [VACC_ChillerSetReq_cnt]
  VACC_PECoolingMode_enum/1 -> [VACC_PECoolingMode_enum]
  OR2/1 -> OR3/1
  [VACC_PECoolingMode_enum] -> Relational Operator1/1
  [VACC_PECoolingMode_enum] -> Relational Operator3/1
  Constant11/1 -> Relational Operator3/2
  Constant10/1 -> Relational Operator1/2
  Relational Operator3/1 -> OR2/1
  Relational Operator1/1 -> OR2/2
  OR3/1 -> Switch2/2
  [VACC_ChillerSetReq_cnt] -> Relational Operator2/1
  Constant1/1 -> Relational Operator2/2
  Relational Operator2/1 -> OR3/2
  Switch2/1 -> VACC_ACReq_enum/1
  Constant2/1 -> Switch2/1
  Constant3/1 -> Switch2/3

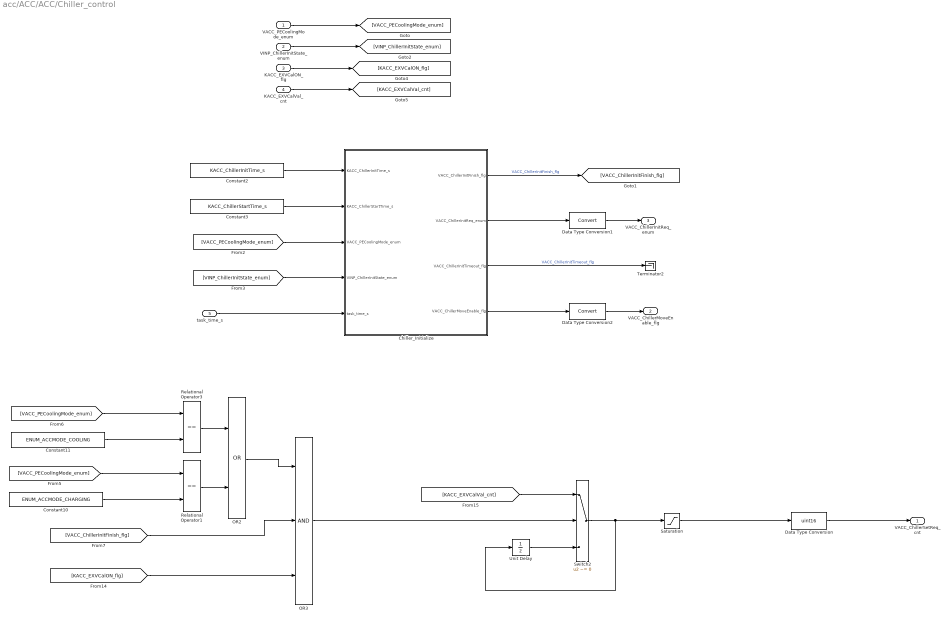
== system acc/ACC/ACC/Chiller_control ==
  VACC_PECoolingMode_enum : Inport
  VINP_ChillerInitState_enum : Inport  Port=2
  KACC_EXVCalON_flg : Inport  Port=3
  KACC_EXVCalVal_cnt : Inport  Port=4
  task_time_s : Inport  Port=5
  Chiller_Initialize : Stateflow chart  TreatAsAtomicUnit=on
  Constant10 : Constant  Value=ENUM_ACCMODE_CHARGING
  Constant11 : Constant  Value=ENUM_ACCMODE_COOLING
  Constant2 : Constant  Value=KACC_ChillerInitTime_s
  Constant3 : Constant  Value=KACC_ChillerStartTime_s
  Data Type Conversion : DataTypeConversion  OutDataTypeStr=uint16
  Data Type Conversion1 : DataTypeConversion
  Data Type Conversion2 : DataTypeConversion
  OR2 : Logic  Operator=OR  AllPortsSameDT=off  OutDataTypeStr=boolean
  OR3 : Logic  Inputs=3  AllPortsSameDT=off  OutDataTypeStr=boolean
  Relational Operator1 : RelationalOperator  Operator===  OutDataTypeStr=boolean  RndMeth=Simplest
  Relational Operator3 : RelationalOperator  Operator===  OutDataTypeStr=boolean  RndMeth=Simplest
  Saturation : Saturate  UpperLimit=576  LowerLimit=0
      settings: AttributesFormatString=|
      | LowerLimi: %<LowerLimit>
      | UpperLimit: %<UpperLimit>
  Switch2 : Switch  Criteria=u2 ~= 0
      settings: AttributesFormatString=%<Criteria>
  Terminator2 : Terminator
  Unit Delay : UnitDelay  SampleTime=-1  HasFrameUpgradeWarning=on
      settings: AttributesFormatString=InitialCondition: %<InitialCondition>
  VACC_ChillerSetReq_cnt : Outport
  VACC_ChillerMoveEnable_flg : Outport  Port=2
  VACC_ChillerInitReq_enum : Outport  Port=3
  wires:
  Chiller_Initialize/4(VACC_ChillerMoveEnable_flg) -> Data Type Conversion2/1
  Data Type Conversion2/1 -> VACC_ChillerMoveEnable_flg/1
  Data Type Conversion1/1 -> VACC_ChillerInitReq_enum/1
  Switch2/1 -> Saturation/1, Unit Delay/1
  Unit Delay/1 -> Switch2/3
  Saturation/1 -> Data Type Conversion/1
  OR3/1 -> Switch2/2
  [KACC_EXVCalON_flg] -> OR3/3
  Chiller_Initialize/3(VACC_ChillerInitTimeout_flg) -> Terminator2/1  "VACC_ChillerInitTimeout_flg"
  Chiller_Initialize/2(VACC_ChillerInitReq_enum) -> Data Type Conversion1/1
  Relational Operator1/1 -> OR2/2
  Relational Operator3/1 -> OR2/1
  Constant10/1 -> Relational Operator1/2
  Constant11/1 -> Relational Operator3/2
  [VACC_PECoolingMode_enum] -> Relational Operator3/1
  [VACC_PECoolingMode_enum] -> Relational Operator1/1
  OR2/1 -> OR3/1
  [VACC_ChillerInitFinish_flg] -> OR3/2
  Data Type Conversion/1 -> VACC_ChillerSetReq_cnt/1
  task_time_s/1 -> Chiller_Initialize/5(task_time_s)
  [VACC_PECoolingMode_enum] -> Chiller_Initialize/3(VACC_PECoolingMode_enum)
  [VINP_ChillerInitState_enum] -> Chiller_Initialize/4(VINP_ChillerInitState_enum)
  Constant3/1 -> Chiller_Initialize/2(KACC_ChillerStartTime_s)
  Constant2/1 -> Chiller_Initialize/1(KACC_ChillerInitTime_s)
  Chiller_Initialize/1(VACC_ChillerInitFinish_flg) -> [VACC_ChillerInitFinish_flg]  "VACC_ChillerInitFinish_flg"
  [KACC_EXVCalVal_cnt] -> Switch2/1
  KACC_EXVCalVal_cnt/1 -> [KACC_EXVCalVal_cnt]
  KACC_EXVCalON_flg/1 -> [KACC_EXVCalON_flg]
  VACC_PECoolingMode_enum/1 -> [VACC_PECoolingMode_enum]
  VINP_ChillerInitState_enum/1 -> [VINP_ChillerInitState_enum]

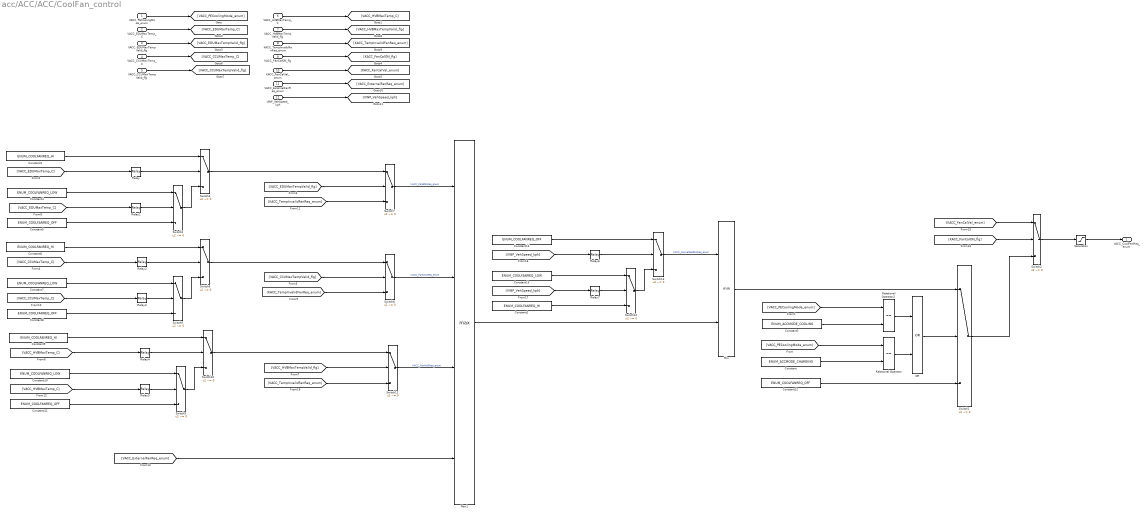
== system acc/ACC/ACC/CoolFan_control ==
  VACC_PECoolingMode_enum : Inport
  VACC_EDUMaxTemp_C : Inport  Port=2
  VACC_EDUMaxTempValid_flg : Inport  Port=3
  VACC_CCUMaxTemp_C : Inport  Port=4
  VACC_CCUMaxTempValid_flg : Inport  Port=5
  VACC_HVBMaxTemp_C : Inport  Port=6
  VACC_HVBMaxTempValid_flg : Inport  Port=7
  KACC_TempInvalidFanReq_enum : Inport  Port=8
  KACC_FanCalON_flg : Inport  Port=9
  KACC_FanCalVal_enum : Inport  Port=10
  VACC_ExternalFanReq_enum : Inport  Port=11
  VINP_VehSpeed_kph : Inport  Port=12
  Constant : Constant  Value=ENUM_ACCMODE_CHARGING
  Constant1 : Constant  Value=ENUM_ACCMODE_COOLING
  Constant{4,7,10,13} (4 alike) : Constant  Value=ENUM_COOLFANREQ_LOW
  Constant{5,8,11..12,14} (5 alike) : Constant  Value=ENUM_COOLFANREQ_OFF
  Constant{2..3,6,9} (4 alike) : Constant  Value=ENUM_COOLFANREQ_HI
  Max1 : MinMax  Function=max  Inputs=4
  Min : MinMax  Inputs=2
  OR : Logic  Operator=OR  AllPortsSameDT=off  OutDataTypeStr=boolean
  Relational Operator : RelationalOperator  Operator===  OutDataTypeStr=boolean  RndMeth=Simplest
  Relational Operator2 : RelationalOperator  Operator===  OutDataTypeStr=boolean  RndMeth=Simplest
  Relay : Relay  OnSwitchValue=KACC_EDUFanHighOnTemp_C  OffSwitchValue=KACC_EDUFanHighOffTemp_C
      settings: AttributesFormatString=|
      | ON: %<OnSwitchValue>
      | OFF: %<OffSwitchValue>
  Relay1 : Relay  OnSwitchValue=KACC_EDUFanLowOnTemp_C  OffSwitchValue=KACC_EDUFanLowOffTemp_C
      settings: AttributesFormatString=|
      | ON: %<OnSwitchValue>
      | OFF: %<OffSwitchValue>
  Relay2 : Relay  OnSwitchValue=KACC_CCUFanHighOnTemp_C  OffSwitchValue=KACC_CCUFanHighOffTemp_C
      settings: AttributesFormatString=|
      | ON: %<OnSwitchValue>
      | OFF: %<OffSwitchValue>
  Relay3 : Relay  OnSwitchValue=KACC_CCUFanLowOnTemp_C  OffSwitchValue=KACC_CCUFanLowOffTemp_C
      settings: AttributesFormatString=|
      | ON: %<OnSwitchValue>
      | OFF: %<OffSwitchValue>
  Relay4 : Relay  OnSwitchValue=KACC_HVBFanHighOnTemp_C  OffSwitchValue=KACC_HVBFanHighOffTemp_C
      settings: AttributesFormatString=|
      | ON: %<OnSwitchValue>
      | OFF: %<OffSwitchValue>
  Relay5 : Relay  OnSwitchValue=KACC_HVBFanLowOnTemp_C  OffSwitchValue=KACC_HVBFanLowOffTemp_C
      settings: AttributesFormatString=|
      | ON: %<OnSwitchValue>
      | OFF: %<OffSwitchValue>
  Relay6 : Relay  OnSwitchValue=KACC_VehSpdFanLowOff_kph  OffSwitchValue=KACC_VehSpdFanLowOn_kph
      settings: AttributesFormatString=|
      | ON: %<OnSwitchValue>
      | OFF: %<OffSwitchValue>
  Relay7 : Relay  OnSwitchValue=KACC_VehSpdFanHighOff_kph  OffSwitchValue=KACC_VehSpdFanHighOn_kph
      settings: AttributesFormatString=|
      | ON: %<OnSwitchValue>
      | OFF: %<OffSwitchValue>
  Saturation : Saturate  UpperLimit=2  LowerLimit=0
      settings: AttributesFormatString=|
      | LowerLimi: %<LowerLimit>
      | UpperLimit: %<UpperLimit>
  Switch{1..13} (13 alike) : Switch  Criteria=u2 ~= 0
      settings: AttributesFormatString=%<Criteria>
  VACC_CoolFanReq_enum : Outport
  wires:
  Min/1 -> Switch1/1
  Switch13/1 -> Min/1  "VACC_FanVehSpdDisReq_enum"
  Max1/1 -> Min/2
  Constant2/1 -> Switch12/3
  [VINP_VehSpeed_kph] -> Relay7/1
  Constant14/1 -> Switch13/1
  [VINP_VehSpeed_kph] -> Relay6/1
  Switch12/1 -> Switch13/3
  Constant13/1 -> Switch12/1
  Relay7/1 -> Switch12/2
  Relay6/1 -> Switch13/2
  Constant12/1 -> Switch1/3
  [VACC_ExternalFanReq_enum] -> Max1/4
  Switch11/1 -> Max1/3  "VACC_FanHVBReq_enum"
  Switch8/1 -> Max1/2  "VACC_FanCCUReq_enum"
  Switch7/1 -> Max1/1  "VACC_FanEDUReq_enum"
  VINP_VehSpeed_kph/1 -> [VINP_VehSpeed_kph]
  [KACC_TempInvalidFanReq_enum] -> Switch11/3
  Switch10/1 -> Switch11/1
  Constant11/1 -> Switch9/3
  Constant10/1 -> Switch9/1
  Relay5/1 -> Switch9/2
  Switch9/1 -> Switch10/3
  Constant9/1 -> Switch10/1
  Relay4/1 -> Switch10/2
  [VACC_HVBMaxTempValid_flg] -> Switch11/2
  [VACC_HVBMaxTemp_C] -> Relay4/1
  [VACC_HVBMaxTemp_C] -> Relay5/1
  [VACC_CCUMaxTemp_C] -> Relay3/1
  [VACC_CCUMaxTemp_C] -> Relay2/1
  [VACC_CCUMaxTempValid_flg] -> Switch8/2
  Relay2/1 -> Switch6/2
  Constant6/1 -> Switch6/1
  Switch5/1 -> Switch6/3
  Relay3/1 -> Switch5/2
  Constant7/1 -> Switch5/1
  Constant8/1 -> Switch5/3
  Switch6/1 -> Switch8/1
  [KACC_TempInvalidFanReq_enum] -> Switch8/3
  [KACC_TempInvalidFanReq_enum] -> Switch7/3
  [VACC_EDUMaxTempValid_flg] -> Switch7/2
  Switch4/1 -> Switch7/1
  Constant5/1 -> Switch3/3
  Constant4/1 -> Switch3/1
  Relay1/1 -> Switch3/2
  [VACC_EDUMaxTemp_C] -> Relay1/1
  Switch3/1 -> Switch4/3
  Constant3/1 -> Switch4/1
  Relay/1 -> Switch4/2
  [VACC_EDUMaxTemp_C] -> Relay/1
  VACC_ExternalFanReq_enum/1 -> [VACC_ExternalFanReq_enum]
  [KACC_FanCalVal_enum] -> Switch2/1
  [KACC_FanCalON_flg] -> Switch2/2
  KACC_FanCalVal_enum/1 -> [KACC_FanCalVal_enum]
  KACC_FanCalON_flg/1 -> [KACC_FanCalON_flg]
  Saturation/1 -> VACC_CoolFanReq_enum/1
  Switch2/1 -> Saturation/1
  VACC_PECoolingMode_enum/1 -> [VACC_PECoolingMode_enum]
  [VACC_PECoolingMode_enum] -> Relational Operator/1
  [VACC_PECoolingMode_enum] -> Relational Operator2/1
  Constant1/1 -> Relational Operator2/2
  Constant/1 -> Relational Operator/2
  Switch1/1 -> Switch2/3
  VACC_HVBMaxTemp_C/1 -> [VACC_HVBMaxTemp_C]
  Relational Operator2/1 -> OR/1
  Relational Operator/1 -> OR/2
  OR/1 -> Switch1/2
  VACC_EDUMaxTemp_C/1 -> [VACC_EDUMaxTemp_C]
  VACC_EDUMaxTempValid_flg/1 -> [VACC_EDUMaxTempValid_flg]
  VACC_CCUMaxTemp_C/1 -> [VACC_CCUMaxTemp_C]
  VACC_CCUMaxTempValid_flg/1 -> [VACC_CCUMaxTempValid_flg]
  VACC_HVBMaxTempValid_flg/1 -> [VACC_HVBMaxTempValid_flg]
  KACC_TempInvalidFanReq_enum/1 -> [KACC_TempInvalidFanReq_enum]

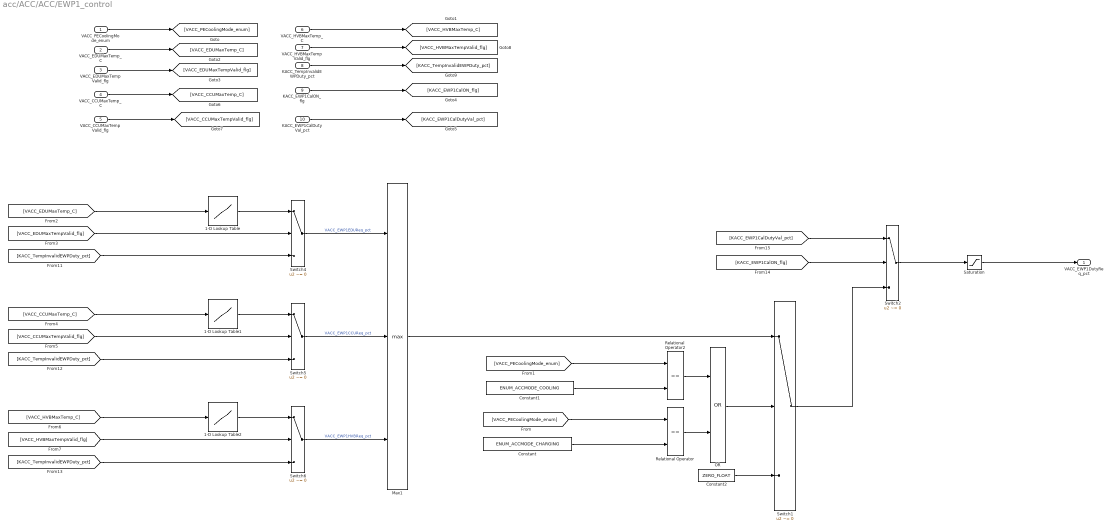
== system acc/ACC/ACC/EWP1_control ==
  VACC_PECoolingMode_enum : Inport
  VACC_EDUMaxTemp_C : Inport  Port=2
  VACC_EDUMaxTempValid_flg : Inport  Port=3
  VACC_CCUMaxTemp_C : Inport  Port=4
  VACC_CCUMaxTempValid_flg : Inport  Port=5
  VACC_HVBMaxTemp_C : Inport  Port=6
  VACC_HVBMaxTempValid_flg : Inport  Port=7
  KACC_TempInvalidEWPDuty_pct : Inport  Port=8
  KACC_EWP1CalON_flg : Inport  Port=9
  KACC_EWP1CalDutyVal_pct : Inport  Port=10
  1-D Lookup Table : Lookup_n-D  NumberOfTableDimensions=1  BreakpointsForDimension1=AACC_EWP1EDUReq_X_C  Table=MACC_EWP1EDUReq_Y_pct  UseLastTableValue=on  InternalRulePriority=Speed  RndMeth=Simplest  InputSameDT=on
  1-D Lookup Table1 : Lookup_n-D  NumberOfTableDimensions=1  BreakpointsForDimension1=AACC_EWP1CCUReq_X_C  Table=MACC_EWP1CCUReq_Y_pct  UseLastTableValue=on  InternalRulePriority=Speed  RndMeth=Simplest  InputSameDT=on
  1-D Lookup Table2 : Lookup_n-D  NumberOfTableDimensions=1  BreakpointsForDimension1=AACC_EWP1HVBReq_X_C  Table=MACC_EWP1HVBReq_Y_pct  UseLastTableValue=on  InternalRulePriority=Speed  RndMeth=Simplest  InputSameDT=on
  Constant : Constant  Value=ENUM_ACCMODE_CHARGING
  Constant1 : Constant  Value=ENUM_ACCMODE_COOLING
  Constant2 : Constant  Value=ZERO_FLOAT
  Max1 : MinMax  Function=max  Inputs=3
  OR : Logic  Operator=OR  AllPortsSameDT=off  OutDataTypeStr=boolean
  Relational Operator : RelationalOperator  Operator===  OutDataTypeStr=boolean  RndMeth=Simplest
  Relational Operator2 : RelationalOperator  Operator===  OutDataTypeStr=boolean  RndMeth=Simplest
  Saturation : Saturate  UpperLimit=100  LowerLimit=0
      settings: AttributesFormatString=|
      | LowerLimi: %<LowerLimit>
      | UpperLimit: %<UpperLimit>
  Switch{1..2,4..6} (5 alike) : Switch  Criteria=u2 ~= 0
      settings: AttributesFormatString=%<Criteria>
  VACC_EWP1DutyReq_pct : Outport
  wires:
  Saturation/1 -> VACC_EWP1DutyReq_pct/1
  [KACC_EWP1CalDutyVal_pct] -> Switch2/1
  [KACC_EWP1CalON_flg] -> Switch2/2
  [KACC_TempInvalidEWPDuty_pct] -> Switch6/3
  [VACC_HVBMaxTemp_C] -> 1-D Lookup Table2/1
  [VACC_HVBMaxTempValid_flg] -> Switch6/2
  1-D Lookup Table2/1 -> Switch6/1
  Switch6/1 -> Max1/3  "VACC_EWP1HVBReq_pct"
  [KACC_TempInvalidEWPDuty_pct] -> Switch5/3
  [VACC_CCUMaxTempValid_flg] -> Switch5/2
  1-D Lookup Table1/1 -> Switch5/1
  [VACC_CCUMaxTemp_C] -> 1-D Lookup Table1/1
  1-D Lookup Table/1 -> Switch4/1
  [VACC_EDUMaxTemp_C] -> 1-D Lookup Table/1
  [KACC_TempInvalidEWPDuty_pct] -> Switch4/3
  [VACC_EDUMaxTempValid_flg] -> Switch4/2
  KACC_EWP1CalDutyVal_pct/1 -> [KACC_EWP1CalDutyVal_pct]
  KACC_EWP1CalON_flg/1 -> [KACC_EWP1CalON_flg]
  Switch2/1 -> Saturation/1
  VACC_PECoolingMode_enum/1 -> [VACC_PECoolingMode_enum]
  [VACC_PECoolingMode_enum] -> Relational Operator/1
  [VACC_PECoolingMode_enum] -> Relational Operator2/1
  Max1/1 -> Switch1/1
  Constant1/1 -> Relational Operator2/2
  Constant/1 -> Relational Operator/2
  Switch1/1 -> Switch2/3
  VACC_HVBMaxTemp_C/1 -> [VACC_HVBMaxTemp_C]
  Relational Operator2/1 -> OR/1
  Relational Operator/1 -> OR/2
  OR/1 -> Switch1/2
  Constant2/1 -> Switch1/3
  VACC_EDUMaxTemp_C/1 -> [VACC_EDUMaxTemp_C]
  VACC_EDUMaxTempValid_flg/1 -> [VACC_EDUMaxTempValid_flg]
  VACC_CCUMaxTemp_C/1 -> [VACC_CCUMaxTemp_C]
  VACC_CCUMaxTempValid_flg/1 -> [VACC_CCUMaxTempValid_flg]
  VACC_HVBMaxTempValid_flg/1 -> [VACC_HVBMaxTempValid_flg]
  KACC_TempInvalidEWPDuty_pct/1 -> [KACC_TempInvalidEWPDuty_pct]
  Switch4/1 -> Max1/1  "VACC_EWP1EDUReq_pct"
  Switch5/1 -> Max1/2  "VACC_EWP1CCUReq_pct"

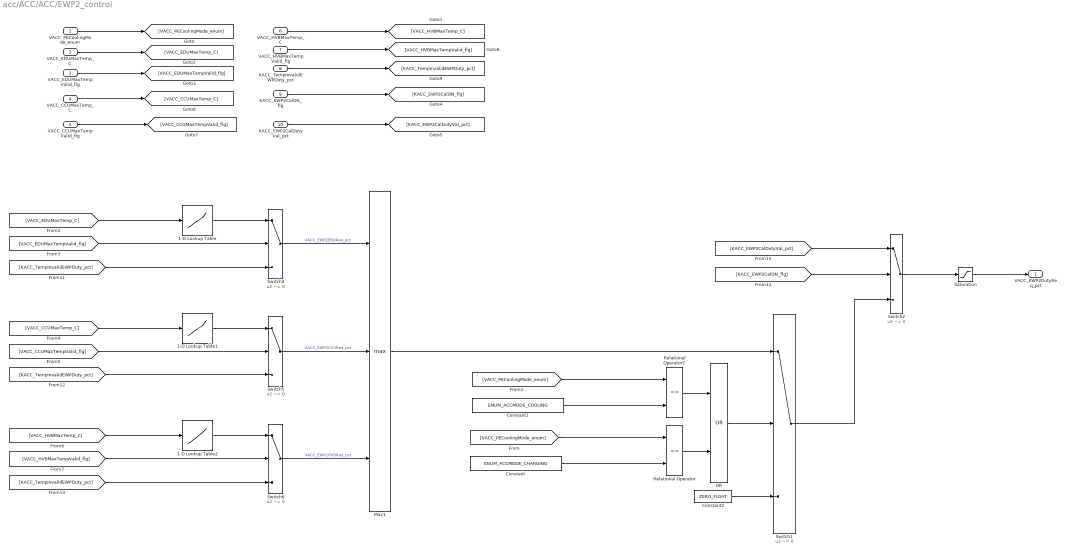
== system acc/ACC/ACC/EWP2_control ==
  VACC_PECoolingMode_enum : Inport
  VACC_EDUMaxTemp_C : Inport  Port=2
  VACC_EDUMaxTempValid_flg : Inport  Port=3
  VACC_CCUMaxTemp_C : Inport  Port=4
  VACC_CCUMaxTempValid_flg : Inport  Port=5
  VACC_HVBMaxTemp_C : Inport  Port=6
  VACC_HVBMaxTempValid_flg : Inport  Port=7
  KACC_TempInvalidEWPDuty_pct : Inport  Port=8
  KACC_EWP2CalON_flg : Inport  Port=9
  KACC_EWP2CalDutyVal_pct : Inport  Port=10
  1-D Lookup Table : Lookup_n-D  NumberOfTableDimensions=1  BreakpointsForDimension1=AACC_EWP2EDUReq_X_C  Table=MACC_EWP2EDUReq_Y_pct  UseLastTableValue=on  InternalRulePriority=Speed  RndMeth=Simplest  InputSameDT=on
  1-D Lookup Table1 : Lookup_n-D  NumberOfTableDimensions=1  BreakpointsForDimension1=AACC_EWP2CCUReq_X_C  Table=MACC_EWP2CCUReq_Y_pct  UseLastTableValue=on  InternalRulePriority=Speed  RndMeth=Simplest  InputSameDT=on
  1-D Lookup Table2 : Lookup_n-D  NumberOfTableDimensions=1  BreakpointsForDimension1=AACC_EWP2HVBReq_X_C  Table=MACC_EWP2HVBReq_Y_pct  UseLastTableValue=on  InternalRulePriority=Speed  RndMeth=Simplest  InputSameDT=on
  Constant : Constant  Value=ENUM_ACCMODE_CHARGING
  Constant1 : Constant  Value=ENUM_ACCMODE_COOLING
  Constant2 : Constant  Value=ZERO_FLOAT
  Max1 : MinMax  Function=max  Inputs=3
  OR : Logic  Operator=OR  AllPortsSameDT=off  OutDataTypeStr=boolean
  Relational Operator : RelationalOperator  Operator===  OutDataTypeStr=boolean  RndMeth=Simplest
  Relational Operator2 : RelationalOperator  Operator===  OutDataTypeStr=boolean  RndMeth=Simplest
  Saturation : Saturate  UpperLimit=100  LowerLimit=0
      settings: AttributesFormatString=|
      | LowerLimi: %<LowerLimit>
      | UpperLimit: %<UpperLimit>
  Switch{1..2,4..6} (5 alike) : Switch  Criteria=u2 ~= 0
      settings: AttributesFormatString=%<Criteria>
  VACC_EWP2DutyReq_pct : Outport
  wires:
  Switch5/1 -> Max1/2  "VACC_EWP2CCUReq_pct"
  Switch4/1 -> Max1/1  "VACC_EWP2EDUReq_pct"
  KACC_TempInvalidEWPDuty_pct/1 -> [KACC_TempInvalidEWPDuty_pct]
  VACC_HVBMaxTempValid_flg/1 -> [VACC_HVBMaxTempValid_flg]
  VACC_CCUMaxTempValid_flg/1 -> [VACC_CCUMaxTempValid_flg]
  VACC_CCUMaxTemp_C/1 -> [VACC_CCUMaxTemp_C]
  VACC_EDUMaxTempValid_flg/1 -> [VACC_EDUMaxTempValid_flg]
  VACC_EDUMaxTemp_C/1 -> [VACC_EDUMaxTemp_C]
  Constant2/1 -> Switch1/3
  OR/1 -> Switch1/2
  Relational Operator/1 -> OR/2
  Relational Operator2/1 -> OR/1
  VACC_HVBMaxTemp_C/1 -> [VACC_HVBMaxTemp_C]
  Switch1/1 -> Switch2/3
  Constant/1 -> Relational Operator/2
  Constant1/1 -> Relational Operator2/2
  Max1/1 -> Switch1/1
  [VACC_PECoolingMode_enum] -> Relational Operator2/1
  [VACC_PECoolingMode_enum] -> Relational Operator/1
  VACC_PECoolingMode_enum/1 -> [VACC_PECoolingMode_enum]
  Switch2/1 -> Saturation/1
  Saturation/1 -> VACC_EWP2DutyReq_pct/1
  KACC_EWP2CalON_flg/1 -> [KACC_EWP2CalON_flg]
  KACC_EWP2CalDutyVal_pct/1 -> [KACC_EWP2CalDutyVal_pct]
  [VACC_EDUMaxTempValid_flg] -> Switch4/2
  [KACC_TempInvalidEWPDuty_pct] -> Switch4/3
  [VACC_EDUMaxTemp_C] -> 1-D Lookup Table/1
  1-D Lookup Table/1 -> Switch4/1
  [VACC_CCUMaxTemp_C] -> 1-D Lookup Table1/1
  1-D Lookup Table1/1 -> Switch5/1
  [VACC_CCUMaxTempValid_flg] -> Switch5/2
  [KACC_TempInvalidEWPDuty_pct] -> Switch5/3
  Switch6/1 -> Max1/3  "VACC_EWP2HVBReq_pct"
  1-D Lookup Table2/1 -> Switch6/1
  [VACC_HVBMaxTempValid_flg] -> Switch6/2
  [VACC_HVBMaxTemp_C] -> 1-D Lookup Table2/1
  [KACC_TempInvalidEWPDuty_pct] -> Switch6/3
  [KACC_EWP2CalON_flg] -> Switch2/2
  [KACC_EWP2CalDutyVal_pct] -> Switch2/1

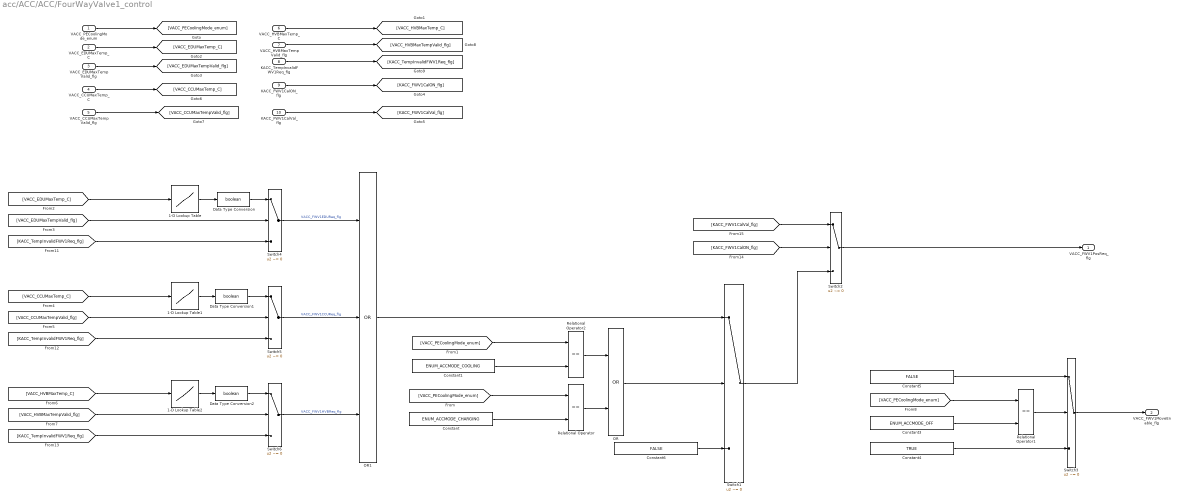
== system acc/ACC/ACC/FourWayValve1_control ==
  VACC_PECoolingMode_enum : Inport
  VACC_EDUMaxTemp_C : Inport  Port=2
  VACC_EDUMaxTempValid_flg : Inport  Port=3
  VACC_CCUMaxTemp_C : Inport  Port=4
  VACC_CCUMaxTempValid_flg : Inport  Port=5
  VACC_HVBMaxTemp_C : Inport  Port=6
  VACC_HVBMaxTempValid_flg : Inport  Port=7
  KACC_TempInvalidFWV1Req_flg : Inport  Port=8
  KACC_FWV1CalON_flg : Inport  Port=9
  KACC_FWV1CalVal_flg : Inport  Port=10
  1-D Lookup Table : Lookup_n-D  NumberOfTableDimensions=1  BreakpointsForDimension1=AACC_FWV1EDUReq_X_C  Table=MACC_FWV1EDUReq_Y_flg  InterpMethod=Flat  UseLastTableValue=on  InternalRulePriority=Speed  RndMeth=Simplest  InputSameDT=on
  1-D Lookup Table1 : Lookup_n-D  NumberOfTableDimensions=1  BreakpointsForDimension1=AACC_FWV1CCUReq_X_C  Table=MACC_FWV1CCUReq_Y_flg  InterpMethod=Flat  UseLastTableValue=on  InternalRulePriority=Speed  RndMeth=Simplest  InputSameDT=on
  1-D Lookup Table2 : Lookup_n-D  NumberOfTableDimensions=1  BreakpointsForDimension1=AACC_FWV1HVBReq_X_C  Table=MACC_FWV1HVBReq_Y_flg  InterpMethod=Flat  UseLastTableValue=on  InternalRulePriority=Speed  RndMeth=Simplest  InputSameDT=on
  Constant : Constant  Value=ENUM_ACCMODE_CHARGING
  Constant1 : Constant  Value=ENUM_ACCMODE_COOLING
  Constant3 : Constant  Value=ENUM_ACCMODE_OFF
  Constant4 : Constant  Value=TRUE
  Constant5 : Constant  Value=FALSE
  Constant6 : Constant  Value=FALSE
  Data Type Conversion : DataTypeConversion  OutDataTypeStr=boolean
  Data Type Conversion1 : DataTypeConversion  OutDataTypeStr=boolean
  Data Type Conversion2 : DataTypeConversion  OutDataTypeStr=boolean
  OR : Logic  Operator=OR  AllPortsSameDT=off  OutDataTypeStr=boolean
  OR1 : Logic  Operator=OR  Inputs=3  AllPortsSameDT=off  OutDataTypeStr=boolean
  Relational Operator : RelationalOperator  Operator===  OutDataTypeStr=boolean  RndMeth=Simplest
  Relational Operator1 : RelationalOperator  Operator===  OutDataTypeStr=boolean  RndMeth=Simplest
  Relational Operator2 : RelationalOperator  Operator===  OutDataTypeStr=boolean  RndMeth=Simplest
  Switch{1..6} (6 alike) : Switch  Criteria=u2 ~= 0
      settings: AttributesFormatString=%<Criteria>
  VACC_FWV1PosReq_flg : Outport
  VACC_FWV1MoveEnable_flg : Outport  Port=2
  wires:
  Data Type Conversion2/1 -> Switch6/1
  Data Type Conversion1/1 -> Switch5/1
  Data Type Conversion/1 -> Switch4/1
  OR1/1 -> Switch1/1
  Constant6/1 -> Switch1/3
  [KACC_FWV1CalVal_flg] -> Switch2/1
  [KACC_FWV1CalON_flg] -> Switch2/2
  [KACC_TempInvalidFWV1Req_flg] -> Switch6/3
  [VACC_HVBMaxTemp_C] -> 1-D Lookup Table2/1
  [VACC_HVBMaxTempValid_flg] -> Switch6/2
  1-D Lookup Table2/1 -> Data Type Conversion2/1
  Switch6/1 -> OR1/3  "VACC_FWV1HVBReq_flg"
  [KACC_TempInvalidFWV1Req_flg] -> Switch5/3
  [VACC_CCUMaxTempValid_flg] -> Switch5/2
  1-D Lookup Table1/1 -> Data Type Conversion1/1
  [VACC_CCUMaxTemp_C] -> 1-D Lookup Table1/1
  1-D Lookup Table/1 -> Data Type Conversion/1
  [VACC_EDUMaxTemp_C] -> 1-D Lookup Table/1
  [KACC_TempInvalidFWV1Req_flg] -> Switch4/3
  [VACC_EDUMaxTempValid_flg] -> Switch4/2
  KACC_FWV1CalVal_flg/1 -> [KACC_FWV1CalVal_flg]
  KACC_FWV1CalON_flg/1 -> [KACC_FWV1CalON_flg]
  Switch2/1 -> VACC_FWV1PosReq_flg/1
  VACC_PECoolingMode_enum/1 -> [VACC_PECoolingMode_enum]
  [VACC_PECoolingMode_enum] -> Relational Operator/1
  [VACC_PECoolingMode_enum] -> Relational Operator2/1
  Constant1/1 -> Relational Operator2/2
  Constant/1 -> Relational Operator/2
  Switch1/1 -> Switch2/3
  VACC_HVBMaxTemp_C/1 -> [VACC_HVBMaxTemp_C]
  Relational Operator2/1 -> OR/1
  Relational Operator/1 -> OR/2
  OR/1 -> Switch1/2
  VACC_EDUMaxTemp_C/1 -> [VACC_EDUMaxTemp_C]
  VACC_EDUMaxTempValid_flg/1 -> [VACC_EDUMaxTempValid_flg]
  VACC_CCUMaxTemp_C/1 -> [VACC_CCUMaxTemp_C]
  VACC_CCUMaxTempValid_flg/1 -> [VACC_CCUMaxTempValid_flg]
  VACC_HVBMaxTempValid_flg/1 -> [VACC_HVBMaxTempValid_flg]
  KACC_TempInvalidFWV1Req_flg/1 -> [KACC_TempInvalidFWV1Req_flg]
  Switch4/1 -> OR1/1  "VACC_FWV1EDUReq_flg"
  Switch5/1 -> OR1/2  "VACC_FWV1CCUReq_flg"
  Constant3/1 -> Relational Operator1/2
  [VACC_PECoolingMode_enum] -> Relational Operator1/1
  Relational Operator1/1 -> Switch3/2
  Switch3/1 -> VACC_FWV1MoveEnable_flg/1
  Constant5/1 -> Switch3/1
  Constant4/1 -> Switch3/3

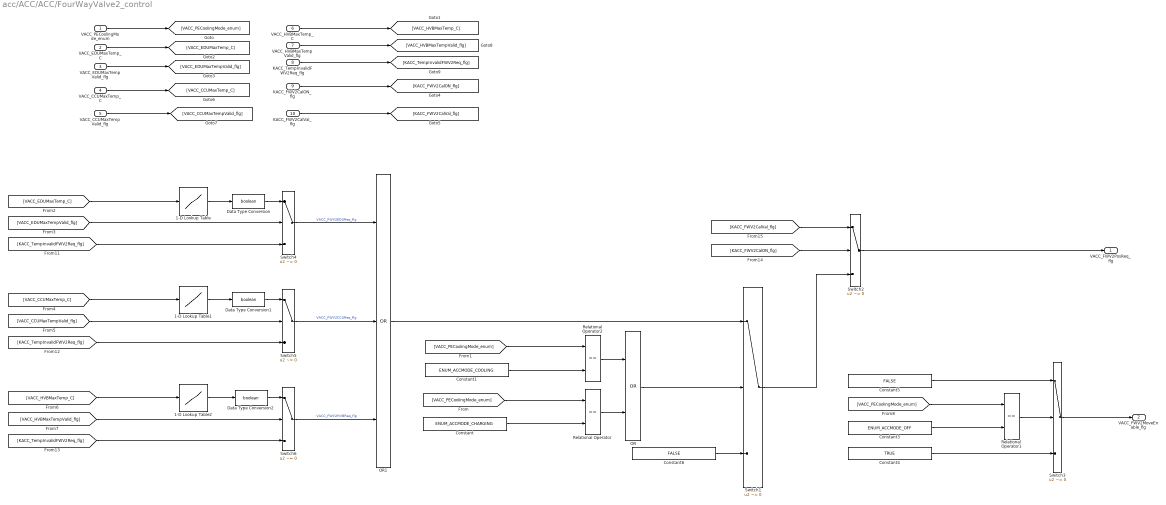
== system acc/ACC/ACC/FourWayValve2_control ==
  VACC_PECoolingMode_enum : Inport
  VACC_EDUMaxTemp_C : Inport  Port=2
  VACC_EDUMaxTempValid_flg : Inport  Port=3
  VACC_CCUMaxTemp_C : Inport  Port=4
  VACC_CCUMaxTempValid_flg : Inport  Port=5
  VACC_HVBMaxTemp_C : Inport  Port=6
  VACC_HVBMaxTempValid_flg : Inport  Port=7
  KACC_TempInvalidFWV2Req_flg : Inport  Port=8
  KACC_FWV2CalON_flg : Inport  Port=9
  KACC_FWV2CalVal_flg : Inport  Port=10
  1-D Lookup Table : Lookup_n-D  NumberOfTableDimensions=1  BreakpointsForDimension1=AACC_FWV2EDUReq_X_C  Table=MACC_FWV2EDUReq_Y_flg  InterpMethod=Flat  UseLastTableValue=on  InternalRulePriority=Speed  RndMeth=Simplest  InputSameDT=on
  1-D Lookup Table1 : Lookup_n-D  NumberOfTableDimensions=1  BreakpointsForDimension1=AACC_FWV2CCUReq_X_C  Table=MACC_FWV2CCUReq_Y_flg  InterpMethod=Flat  UseLastTableValue=on  InternalRulePriority=Speed  RndMeth=Simplest  InputSameDT=on
  1-D Lookup Table2 : Lookup_n-D  NumberOfTableDimensions=1  BreakpointsForDimension1=AACC_FWV2HVBReq_X_C  Table=MACC_FWV2HVBReq_Y_flg  InterpMethod=Flat  UseLastTableValue=on  InternalRulePriority=Speed  RndMeth=Simplest  InputSameDT=on
  Constant : Constant  Value=ENUM_ACCMODE_CHARGING
  Constant1 : Constant  Value=ENUM_ACCMODE_COOLING
  Constant3 : Constant  Value=ENUM_ACCMODE_OFF
  Constant4 : Constant  Value=TRUE
  Constant5 : Constant  Value=FALSE
  Constant6 : Constant  Value=FALSE
  Data Type Conversion : DataTypeConversion  OutDataTypeStr=boolean
  Data Type Conversion1 : DataTypeConversion  OutDataTypeStr=boolean
  Data Type Conversion2 : DataTypeConversion  OutDataTypeStr=boolean
  OR : Logic  Operator=OR  AllPortsSameDT=off  OutDataTypeStr=boolean
  OR1 : Logic  Operator=OR  Inputs=3  AllPortsSameDT=off  OutDataTypeStr=boolean
  Relational Operator : RelationalOperator  Operator===  OutDataTypeStr=boolean  RndMeth=Simplest
  Relational Operator1 : RelationalOperator  Operator===  OutDataTypeStr=boolean  RndMeth=Simplest
  Relational Operator2 : RelationalOperator  Operator===  OutDataTypeStr=boolean  RndMeth=Simplest
  Switch{1..6} (6 alike) : Switch  Criteria=u2 ~= 0
      settings: AttributesFormatString=%<Criteria>
  VACC_FWV2PosReq_flg : Outport
  VACC_FWV2MoveEnable_flg : Outport  Port=2
  wires:
  Data Type Conversion2/1 -> Switch6/1
  Data Type Conversion1/1 -> Switch5/1
  Data Type Conversion/1 -> Switch4/1
  Constant4/1 -> Switch3/3
  Constant5/1 -> Switch3/1
  Switch3/1 -> VACC_FWV2MoveEnable_flg/1
  Relational Operator1/1 -> Switch3/2
  [VACC_PECoolingMode_enum] -> Relational Operator1/1
  Constant3/1 -> Relational Operator1/2
  Switch5/1 -> OR1/2  "VACC_FWV2CCUReq_flg"
  Switch4/1 -> OR1/1  "VACC_FWV2EDUReq_flg"
  KACC_TempInvalidFWV2Req_flg/1 -> [KACC_TempInvalidFWV2Req_flg]
  VACC_HVBMaxTempValid_flg/1 -> [VACC_HVBMaxTempValid_flg]
  VACC_CCUMaxTempValid_flg/1 -> [VACC_CCUMaxTempValid_flg]
  VACC_CCUMaxTemp_C/1 -> [VACC_CCUMaxTemp_C]
  VACC_EDUMaxTempValid_flg/1 -> [VACC_EDUMaxTempValid_flg]
  VACC_EDUMaxTemp_C/1 -> [VACC_EDUMaxTemp_C]
  OR/1 -> Switch1/2
  Relational Operator/1 -> OR/2
  Relational Operator2/1 -> OR/1
  VACC_HVBMaxTemp_C/1 -> [VACC_HVBMaxTemp_C]
  Switch1/1 -> Switch2/3
  Constant/1 -> Relational Operator/2
  Constant1/1 -> Relational Operator2/2
  [VACC_PECoolingMode_enum] -> Relational Operator2/1
  [VACC_PECoolingMode_enum] -> Relational Operator/1
  VACC_PECoolingMode_enum/1 -> [VACC_PECoolingMode_enum]
  Switch2/1 -> VACC_FWV2PosReq_flg/1
  KACC_FWV2CalON_flg/1 -> [KACC_FWV2CalON_flg]
  KACC_FWV2CalVal_flg/1 -> [KACC_FWV2CalVal_flg]
  [VACC_EDUMaxTempValid_flg] -> Switch4/2
  [KACC_TempInvalidFWV2Req_flg] -> Switch4/3
  [VACC_EDUMaxTemp_C] -> 1-D Lookup Table/1
  1-D Lookup Table/1 -> Data Type Conversion/1
  [VACC_CCUMaxTemp_C] -> 1-D Lookup Table1/1
  1-D Lookup Table1/1 -> Data Type Conversion1/1
  [VACC_CCUMaxTempValid_flg] -> Switch5/2
  [KACC_TempInvalidFWV2Req_flg] -> Switch5/3
  Switch6/1 -> OR1/3  "VACC_FWV2HVBReq_flg"
  1-D Lookup Table2/1 -> Data Type Conversion2/1
  [VACC_HVBMaxTempValid_flg] -> Switch6/2
  [VACC_HVBMaxTemp_C] -> 1-D Lookup Table2/1
  [KACC_TempInvalidFWV2Req_flg] -> Switch6/3
  [KACC_FWV2CalON_flg] -> Switch2/2
  [KACC_FWV2CalVal_flg] -> Switch2/1
  Constant6/1 -> Switch1/3
  OR1/1 -> Switch1/1
